simulink model "mpcSetpointQuadprogNoOffset"  (Simulink 8.4)
settings: Solver=ode4  StartTime=0.0  StopTime=200  RelTol=1e-3
undefined symbols (not defined in the file or in its folder): A, b, B, bd, bx, C, dt, g, gt, H, hc, hx, m, n, P, qpopts, quadprog, T
libraries: simulink x1
settings Model: Creator=aeagr  LastModifiedBy=Arthur
settings DebuggingCC: StrictBusMsg=Warning

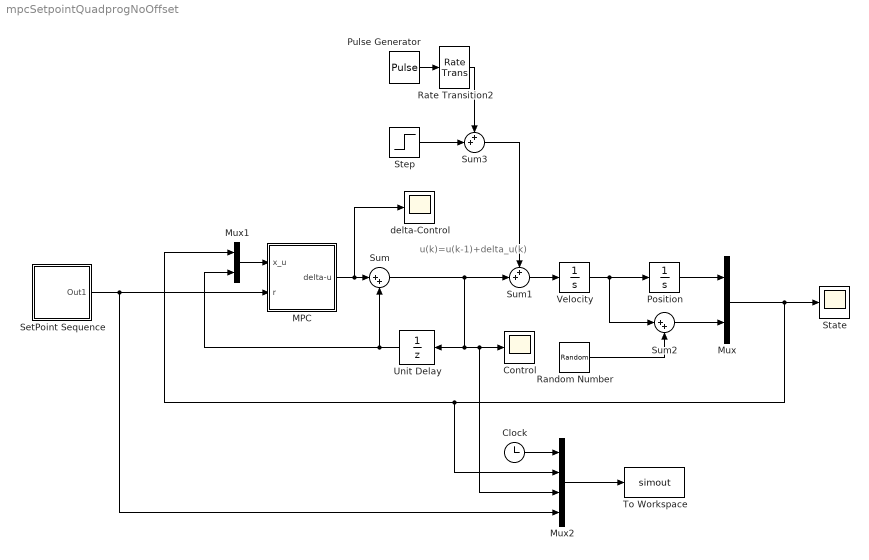
== system mpcSetpointQuadprogNoOffset ==
  note: u(k)=u(k-1)+delta_u(k)
  Clock : Clock
  Control : Scope
      settings: TimeRange=240  YMin=-0.4  YMax=0.35
  MPC : Subsystem  TreatAsAtomicUnit=on  SystemSampleTime=dt
  Mux : Mux  Inputs=2
  Mux1 : Mux  Inputs=2
  Mux2 : Mux
  Position : Integrator
  Pulse Generator : DiscretePulseGenerator  PulseType=Time based  Amplitude=0.1  Period=200  PhaseDelay=101
  Random Number : RandomNumber  Variance=0.000000001*0  SampleTime=dt
  Rate Transition2 : RateTransition
  SetPoint Sequence : Subsystem
  State : Scope
      settings: TimeRange=200  YMin=-0.3  YMax=1
  Step : Step  Time=100  After=0.01*0  SampleTime=0
  Sum : Sum  Inputs=|++
  Sum1 : Sum  Inputs=++|
  Sum2 : Sum  Inputs=|++
  Sum3 : Sum  Inputs=++|
  To Workspace : ToWorkspace  VariableName=simout  SampleTime=-1
  Unit Delay : UnitDelay  SampleTime=dt
  Velocity : Integrator
  delta-Control : Scope
      settings: TimeRange=240  YMin=-0.4  YMax=0.35  SaveName=ScopeData2
  wires:
  Velocity/1 -> Position/1, Sum2/1
  Mux/1 -> State/1, Mux2/2, Mux1/1
  Position/1 -> Mux/1
  SetPoint Sequence/1(Out1) -> Mux2/4, MPC/2(r)
  Sum/1 -> Unit Delay/1, Control/1, Mux2/3, Sum1/2
  Unit Delay/1 -> Sum/2, Mux1/2
  MPC/1(delta-u) -> Sum/1, delta-Control/1
  Mux1/1 -> MPC/1(x_u)
  Sum1/1 -> Velocity/1
  Mux2/1 -> To Workspace/1
  Clock/1 -> Mux2/1
  Step/1 -> Sum3/2
  Pulse Generator/1 -> Rate Transition2/1
  Rate Transition2/1 -> Sum3/1
  Sum3/1 -> Sum1/1
  Sum2/1 -> Mux/2
  Random Number/1 -> Sum2/2

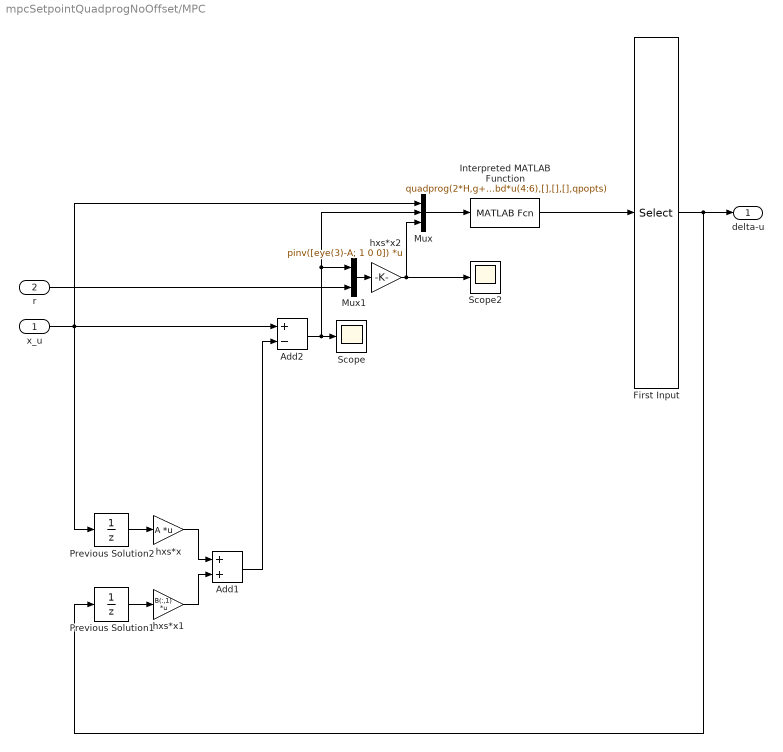
== system mpcSetpointQuadprogNoOffset/MPC ==
  x_u : Inport
  r : Inport  Port=2
  Add1 : Sum
  Add2 : Sum  Inputs=+-
  First Input : Selector  InputPortWidth=T*(n+m)
  Interpreted MATLAB Function : MATLABFcn  MATLABFcn=quadprog(2*H,g+gt*u(7:9),P,hx*u(1:3)+hc,C,b+bx*u(1:3)+bd*u(4:6),[],[],[],qpopts)
  Mux : Mux  Inputs=3
  Mux1 : Mux  Inputs=2
  Previous Solution1 : UnitDelay  SampleTime=-1
  Previous Solution2 : UnitDelay  InitialCondition=[0 0 0]  SampleTime=-1
  Scope : Scope
      settings: YMin=0  YMax=0.00275  SaveName=ScopeData3
  Scope2 : Scope
      settings: YMin=0  YMax=0.00275  SaveName=ScopeData5
  hxs*x : Gain  Gain=A  Multiplication=Matrix(K*u)
  hxs*x1 : Gain  Gain=B(:,1)  Multiplication=Matrix(K*u)
  hxs*x2 : Gain  Gain=pinv([eye(3)-A; 1 0 0])  Multiplication=Matrix(K*u)
  delta-u : Outport
  wires:
  First Input/1 -> delta-u/1, Previous Solution1/1
  Interpreted MATLAB Function/1 -> First Input/1
  x_u/1 -> Previous Solution2/1, Add2/1, Mux/1
  hxs*x/1 -> Add1/1
  Previous Solution1/1 -> hxs*x1/1
  Add1/1 -> Add2/2
  Previous Solution2/1 -> hxs*x/1
  hxs*x1/1 -> Add1/2
  Mux/1 -> Interpreted MATLAB Function/1
  Add2/1 -> Scope/1, Mux/2, Mux1/1
  r/1 -> Mux1/2
  Mux1/1 -> hxs*x2/1
  hxs*x2/1 -> Scope2/1, Mux/3

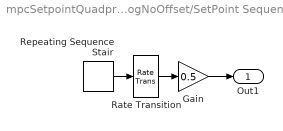
== system mpcSetpointQuadprogNoOffset/SetPoint Sequence ==
  Gain : Gain  Gain=0.5
  Rate Transition : RateTransition
  Repeating Sequence Stair : simulink/Sources/Repeating Sequence Stair  OutValues=[1 0 2 0 3 0 4 0 5 0 6 0].'  tsamp=20  OutMin=[]  OutMax=[]  OutDataTypeStr=double  OutputDataTypeScalingMode=Specify via dialog  OutDataType=double  ConRadixGroup=Best Precision: Vector-wise  OutScaling=2^-12
  Out1 : Outport
  wires:
  Repeating Sequence Stair/1 -> Rate Transition/1
  Rate Transition/1 -> Gain/1
  Gain/1 -> Out1/1
